simulink model "model_state_machine"  (R2024a)
settings: Solver=VariableStepAuto  StartTime=0.0  StopTime=10.0  RelTol=1e-3
settings Model: Creator=Gabriel  LastModifiedBy=Gabriel

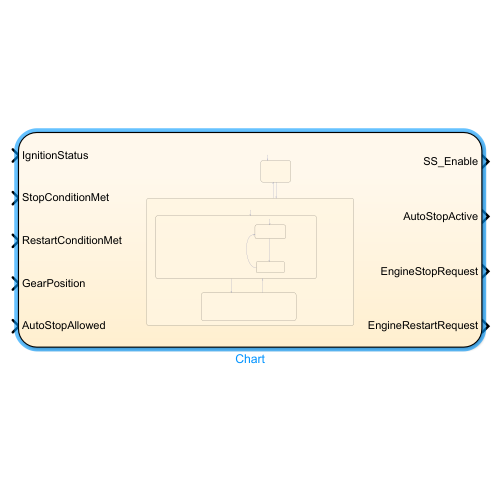
[thumbnail: Simulink's stored preview of the top-level diagram]
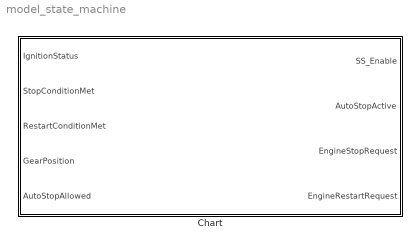
== system model_state_machine ==
  Chart : Stateflow chart  TreatAsAtomicUnit=on

== stateflow chart model_state_machine/Chart ==
  state VehicleOff
    entry:
    SS_Enable = false;
    AutoStopActive =  false;
    EngineStopRequest = false;
    EngineRestartRequest =  false;
  state VehicleOn
    state SS_Available
      state EngineRunning
        entry:
        AutoStopActive = false;
        EngineStopRequest = false;
      state AutoStopActive
        entry:
        AutoStopActive = true;
        EngineRestartRequest = false;
      (default) -> EngineRunning
      AutoStopActive -> EngineRunning : [RestartConditionMet || GearPosition ~= 2 || after(180, sec)]{EngineRestartRequest = true;}
      EngineRunning -> AutoStopActive : [StopConditionMet]{EngineStopRequest = true;}
    state SS_Unavailable
      entry:
      AutoStopActive = false;
      EngineStopRequest = false;
      EngineRestartRequest = false;
    (default) -> SS_Available
    SS_Available -> SS_Unavailable : [SS_Enable == false]
    SS_Unavailable -> SS_Available : [SS_Enable == true]
  (default) -> VehicleOff
  VehicleOn -> VehicleOff : [IgnitionStatus ==  false]
  VehicleOff -> VehicleOn : [IgnitionStatus == true]{SS_Enable = true;}
  data: SS_Enable output; IgnitionStatus input; StopConditionMet input; AutoStopActive output; RestartConditionMet input; EngineStopRequest output; EngineRestartRequest output; GearPosition input; AutoStopAllowed input
